simulink model "controllore_stabilizzante"  (R2026a)
settings: Solver=VariableStepAuto
values from neighbouring files (symbols this model uses):
  A = [0 0 1 0; 0 0 0 1; -2.517 0 -10.915 0; 0 0 0 0]    [sistema_lineare.m]
  B = [0 0; 0 0; 21.83 0; 0 1.236]    [sistema_lineare.m]
  C = [1 0 0 0; 0 1 0 0; 0 0 1 0; 0 0 0 1]    [sistema_lineare.m]
  D = [0 0; 0 0; 0 0; 0 0]    [sistema_lineare.m]
  K = place(A, B, poli_contr)    [K_pole_placement.m]
settings Model: Creator=user  LastModifiedBy=user

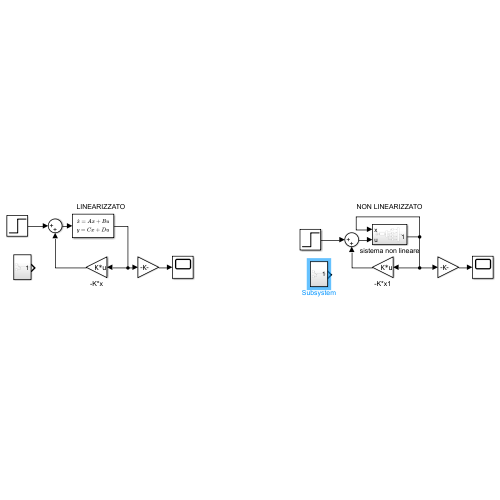
[thumbnail: Simulink's stored preview of the top-level diagram]
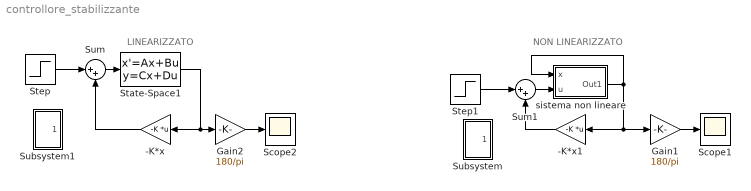
== system controllore_stabilizzante ==
  note: LINEARIZZATO
  note: NON LINEARIZZATO
  -K*x : Gain  Gain=-K  Multiplication=Matrix(K*u)
  -K*x1 : Gain  Gain=-K  Multiplication=Matrix(K*u)
  Gain1 : Gain  Gain=180/pi
  Gain2 : Gain  Gain=180/pi
  Scope1 : Scope
      settings: Title=angoli e velocità angolari  ActiveDisplayYMinimum=-35.4911  ActiveDisplayYMaximum=117.81356  YLabel=stati
  Scope2 : Scope
      settings: Title=angoli e velocità angolari  ActiveDisplayYMinimum=-35.4911  ActiveDisplayYMaximum=117.81356  YLabel=stati
  State-Space1 : StateSpace  A=A  B=B  C=C  D=D  InitialCondition=[1.55;pi/4;0;0]
  Step : Step  Time=5  SampleTime=0
  Step1 : Step  Time=5  SampleTime=0
  Subsystem : Subsystem
  Subsystem1 : Subsystem
  Sum : Sum  Inputs=|++
  Sum1 : Sum  Inputs=|++
  sistema non lineare : Subsystem
  wires:
  State-Space1/1 -> Gain2/1, -K*x/1
  Gain2/1 -> Scope2/1
  Gain1/1 -> Scope1/1
  sistema non lineare/1(Out1) -> sistema non lineare/1(x), Gain1/1, -K*x1/1
  Sum/1 -> State-Space1/1
  -K*x/1 -> Sum/2
  -K*x1/1 -> Sum1/2
  Sum1/1 -> sistema non lineare/2(u)
  Step/1 -> Sum/1
  Step1/1 -> Sum1/1

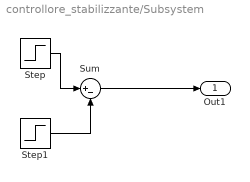
== system controllore_stabilizzante/Subsystem ==
  Step : Step  Time=5  SampleTime=0
  Step1 : Step  Time=5.1  SampleTime=0
  Sum : Sum  Inputs=|+-
  Out1 : Outport
  wires:
  Step/1 -> Sum/1
  Step1/1 -> Sum/2
  Sum/1 -> Out1/1

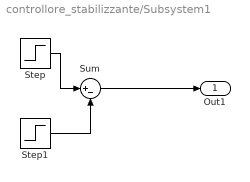
== system controllore_stabilizzante/Subsystem1 ==
  Step : Step  Time=5  SampleTime=0
  Step1 : Step  Time=5.1  SampleTime=0
  Sum : Sum  Inputs=|+-
  Out1 : Outport
  wires:
  Step/1 -> Sum/1
  Step1/1 -> Sum/2
  Sum/1 -> Out1/1

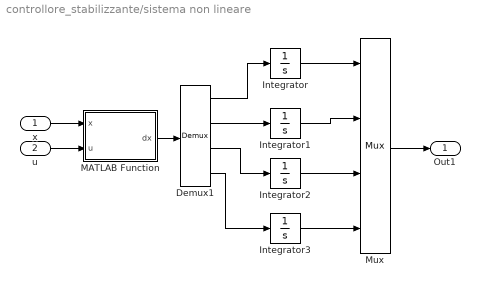
== system controllore_stabilizzante/sistema non lineare ==
  x : Inport
  u : Inport  Port=2
  Demux1 : Demux
  Integrator : Integrator  InitialCondition=1.55
  Integrator1 : Integrator  InitialCondition=pi/4
  Integrator2 : Integrator
  Integrator3 : Integrator
  MATLAB Function : MATLAB Function  TreatAsAtomicUnit=on
  Mux : Mux
  Out1 : Outport  PortDimensions=4
  wires:
  MATLAB Function/1(dx) -> Demux1/1
  Demux1/1 -> Integrator/1
  Demux1/2 -> Integrator1/1
  Mux/1 -> Out1/1
  x/1 -> MATLAB Function/1(x)
  u/1 -> MATLAB Function/2(u)
  Integrator/1 -> Mux/1
  Integrator1/1 -> Mux/2
  Integrator3/1 -> Mux/4
  Integrator2/1 -> Mux/3
  Demux1/3 -> Integrator2/1
  Demux1/4 -> Integrator3/1

== matlab function controllore_stabilizzante/sistema non lineare/MATLAB Function ==
  data: x input; u input; dx output
function dx = trms_dynamics(x, u)
    % Estrazione degli stati dal vettore x
    x1 = x(1);
    x2 = x(2);
    x3 = x(3);
    x4 = x(4);
    
    % Estrazione degli ingressi dal vettore u
    u1 = u(1);
    u2 = u(2);
    
    % Calcolo delle equazioni differenziali
    dx1 = x3;
    dx2 = x4;
    
    % Dinamica di x3
    dx3 = 21.83 * (0.0981*cos(x1) - 0.833*sin(x1) + u1 - 0.195*(x4^2)*sin(x1)*cos(x1) - 0.5*x3);
    
    % Dinamica di x4 (divisa in numeratore e denominatore per chiarezza)
    num_dx4 = u2*cos(x1) - 0.01*x4;
    den_dx4 = 0.01667*(sin(x1)^2) + 0.03728*(cos(x1)^2) + 0.00015;
    dx4 = num_dx4 / den_dx4;
    
    % Vettore colonna delle derivate
    dx = [dx1; dx2; dx3; dx4];
end
